simulink model "MHILSimHWImpl"  (R2024a)
settings: Solver=FixedStepDiscrete  StartTime=0.0  StopTime=2e-4  FixedStep=4e-9  RelTol=1e-3
values from neighbouring files (symbols this model uses):
  cfg = tddbl_model    [HILSimModel.m]
undefined symbols (not defined in the file or in its folder): AXI4, dt, hw, ip, Lite, xc7z020clg400
libraries: hdlBasic x1497, hdlUtilities x3, vmcUtilities x1
(part 1 of 11)
settings Model: Creator=berndorfer
settings DebuggingCC: UnconnectedInputMsg=warning  UnconnectedOutputMsg=warning  UnconnectedLineMsg=warning
settings ModelReferenceCC: EnableRefExpFcnMdlSchedulingChecks=on
settings RTWCC: GPUComputeCapability=3.5  DLArmComputeVersion=19.05

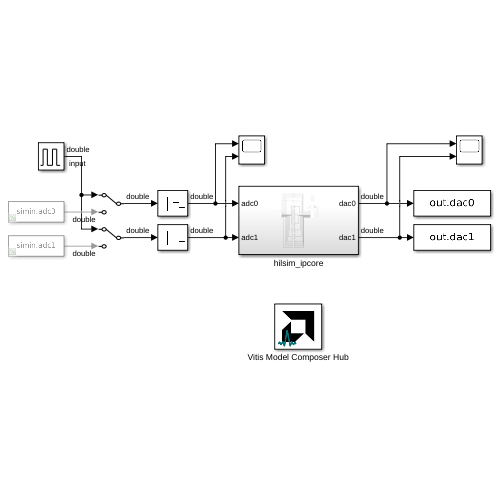
[thumbnail: Simulink's stored preview of the top-level diagram]
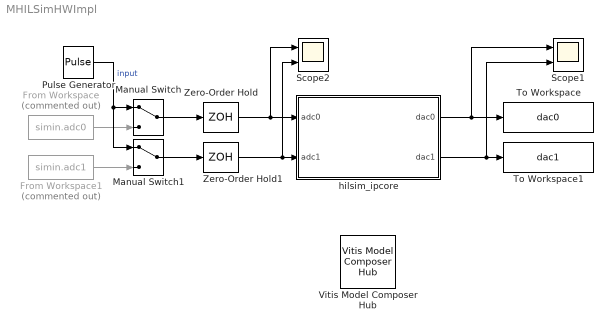
== system MHILSimHWImpl ==
  From Workspace : FromWorkspace  Commented=on  VariableName=simin.adc0
  From Workspace1 : FromWorkspace  Commented=on  VariableName=simin.adc1
  Manual Switch : ManualSwitch
  Manual Switch1 : ManualSwitch
  Pulse Generator : DiscretePulseGenerator  PulseType=Time based  Amplitude=-1  Period=2e-3  PulseWidth=4  PhaseDelay=0.05e-3
  Scope1 : Scope  NumInputPorts=2
  Scope2 : Scope  NumInputPorts=2
  To Workspace : ToWorkspace  VariableName=dac0  SaveFormat=Timeseries  SampleTime=-1
  To Workspace1 : ToWorkspace  VariableName=dac1  SaveFormat=Timeseries  SampleTime=-1
  Vitis Model Composer Hub : vmcUtilities/Vitis Model Composer Hub  Tag=genX  CodeGeneration=off  SubsystemName=hilsim_ipcore  CompilationType=HDLCompilation  SubsystemType=HDLNode  ExportTypeV2=IP Catalog  StartColumn=1  NumberOfColumns=1  TargetDirectory=./code  exportDesign=on  analyzeDesign=off  validateDesignOnHw=off  ExportType=HDL  IpVendor=xilinx.com  IpLibrary=hls  IpVersion=1.0  IpHWLanguage=Verilog  AieCompilerOptions={}  AieSimulatorOptions={}  CreateTestbench=off  TestbenchStackSize=10  RunRtlSim=off  RunCSim=off  RunAieSim=off  AieSimTimeout=50000  RunAieSimProfiling=off  LaunchVitisAnalyzer=off  PlotOutput=off  RunX86Sim=off  X86SimTimeout=10  GenHwImage=off  GenLibadfXo=on  GenHwValidationCode=off  PlatformType=Not Specified  HwSystemType=Baremetal  HwValidationTarget=hw  ProjDevice=xc7z020clg400-1  ProjDevicePart=xc7z020clg400-1  AIEType=None  SamplePeriod=-1  ClockFrequency=200  DataPathParallelism=1  xilinxfamily=zynq  part=xc7z020  speed=-1  package=clg400  directory=./code/ip/hilsim_ipcore/src  testbench=off  incr_netlist=off  synthesis_tool=Vivado  clock_wrapper=Clock Enables  dbl_ovrd=According to Block Masks  dcm_input_clock_period=10  sysclk_period=hw.t_axi_ns  simulink_period=hw.t_axi  eval_field=0  IPInfoJsonString="{\"DUTSubsystemName\":\"hilsim_ipcore\",\"HDLSubsystem\":{\"SubsystemName\":\"hilsim_ipcore\",\"IPName\":\"hilsim_ipcore\",\"IPLibrary\":\"VMC\",\"IPVendor\":\"User Company\",\"IPVersion\":\"1.0\",\"TargetDirectory\":\"./code\",\"SubsystemDir\":\"./code/ip/hilsim_ipcore\",\"FreqHz\":\"125000000\"},\"SubsystemTag\":\"HDLNode\"}"  LogFileName=/home/user/host_home/work/acin/redpitaya-hil-simulator/matlab/hilsim_lib/code/model_composer.log  NThreads=4  IPConfigFile=/tmp/vmctmp-user/10/ipconfig.json
  Zero-Order Hold : ZeroOrderHold  SampleTime=hw.t_s
  Zero-Order Hold1 : ZeroOrderHold  SampleTime=hw.t_s
  hilsim_ipcore : Subsystem
  wires:
  Zero-Order Hold1/1 -> Scope2/2, hilsim_ipcore/2(adc1)
  Zero-Order Hold/1 -> Scope2/1, hilsim_ipcore/1(adc0)
  hilsim_ipcore/1(dac0) -> To Workspace/1, Scope1/1
  hilsim_ipcore/2(dac1) -> To Workspace1/1, Scope1/2
  From Workspace/1 -> Manual Switch/2
  From Workspace1/1 -> Manual Switch1/2
  Manual Switch/1 -> Zero-Order Hold/1
  Manual Switch1/1 -> Zero-Order Hold1/1
  Pulse Generator/1 -> Manual Switch1/1, Manual Switch/1  "input"

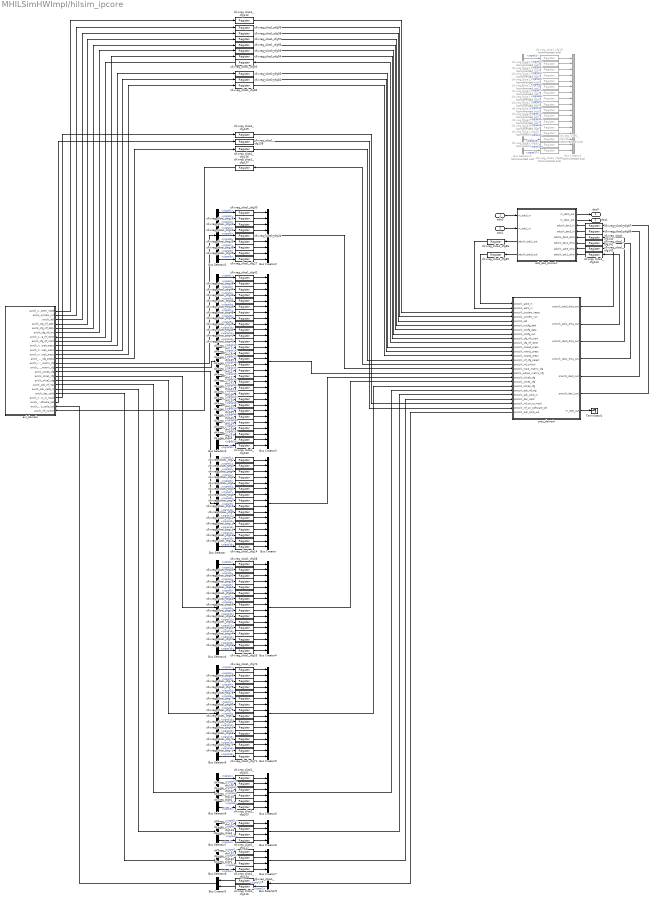
== system MHILSimHWImpl/hilsim_ipcore ==
  adc0 : Inport
  adc1 : Inport  Port=2
  Bus Creator : BusCreator  Inputs=16
  Bus Creator1 : BusCreator  Commented=on  Inputs=17
  Bus Creator2 : BusCreator  Inputs=9
  Bus Creator3 : BusCreator  Inputs=30
  Bus Creator4 : BusCreator  Inputs=16
  Bus Creator5 : BusCreator  Inputs=16
  Bus Creator6 : BusCreator  Inputs=6
  Bus Creator7 : BusCreator  Inputs=4
  Bus Creator8 : BusCreator  Inputs=4
  Bus Creator9 : BusCreator  Inputs=2
  Bus Selector : BusSelector  OutputSignals=signal1,signal2,signal3,signal4,signal5,signal6,signal7,signal8,signal9,signal10,signal11,signal12,signal13,signal14,signal15,signal16
  Bus Selector1 : BusSelector  Commented=on  OutputSignals=signal1,signal2,signal3,signal4,signal5,signal6,signal7,signal8,signal9,signal10,signal11,signal12,signal13,signal14,signal15,signal16,signal17
  Bus Selector2 : BusSelector  OutputSignals=signal1,signal2,signal3,signal4,signal5,signal6,signal7,signal8,signal9
  Bus Selector3 : BusSelector  OutputSignals=signal1,signal2,signal3,signal4,signal5,signal6,signal7,signal8,signal9,signal10,signal11,signal12,signal13,signal14,signal15,signal16,signal17,signal18,signal19,signal20,signal21,signal22,signal23,signal24,signal25,signal26,signal27,signal28,signal29,signal30
  Bus Selector4 : BusSelector  OutputSignals=signal1,signal2,signal3,signal4,signal5,signal6,signal7,signal8,signal9,signal10,signal11,signal12,signal13,signal14,signal15,signal16
  Bus Selector5 : BusSelector  OutputSignals=signal1,signal2,signal3,signal4,signal5,signal6,signal7,signal8,signal9,signal10,signal11,signal12,signal13,signal14,signal15,signal16
  Bus Selector6 : BusSelector  OutputSignals=signal1,signal2,signal3,signal4,signal5,signal6
  Bus Selector7 : BusSelector  OutputSignals=signal1,signal2,signal3,signal4
  Bus Selector8 : BusSelector  OutputSignals=signal1,signal2,signal3,signal4
  Bus Selector9 : BusSelector  OutputSignals=signal1,signal2
  Terminator2 : Terminator
  adc_dac_domain : Subsystem
      settings: PortSchema="{\"entries\":[{\"content\":{\"sides\":[{\"content\":{\"connectorIds\":[\"In1\",\"In2\",\"Out3\",\"Out4\"]},\"type\":\"ConnectorPlacement.EquallySpacedRectSide\",\"uuid\":\"3b4b5965-55e8-468b-ba12-10c3668eb49b\"},{\"content\":{\"connectorIds\":[\"Out1\",\"Out2\",\"In3\",\"In4\",\"In5\",\"In6\",\"In7\",\"In8\"],\"side\":\"RIGHT\"},\"type\":\"ConnectorPlacement.EquallySpacedRectSide\",\"uuid\":\"8bb04938-2ca8-45f3-b211-bd7f875fa19c\"},{\"content\":{\"connectorIds\":[],\"side\":\"TOP\"},\"type\":\"ConnectorPlacement.EquallySpacedRectSide\",\"uuid\":\"4c0cee75-ec1a-4ac7-a2fb-85dd83502d34\"}]},\"type\":\"ConnectorPlacement.EquallySpacedConnector\",\"uuid\":\"be0807c7-02a6-41b2-91cb-ef8260a22db3\"}],\"packageUris\":[\"http://schema.mathworks.com/mf0/Connector/R2020b\"],\"version\":\"1.0\"}"
  axi_domain : Subsystem
      settings: PortSchema="{\"entries\":[{\"content\":{\"sides\":[{\"content\":{\"connectorIds\":[]},\"type\":\"ConnectorPlacement.EquallySpacedRectSide\",\"uuid\":\"0fb9306b-ba57-4fb3-868e-1f06c1028522\"},{\"content\":{\"connectorIds\":[\"Out1\",\"Out2\",\"Out3\",\"Out4\",\"Out5\",\"Out6\",\"In1\",\"Out7\",\"Out8\",\"Out9\",\"Out10\",\"Out11\",\"Out12\",\"Out13\",\"Out14\",\"Out15\",\"Out16\",\"Out17\",\"Out18\",\"Out19\",\"Out20\",\"Out21\",\"In2\",\"In3\"],\"side\":\"RIGHT\"},\"type\":\"ConnectorPlacement.EquallySpacedRectSide\",\"uuid\":\"1b75b5fd-5ede-4f54-9992-e4e539862811\"},{\"content\":{\"connectorIds\":[],\"side\":\"TOP\"},\"type\":\"ConnectorPlacement.EquallySpacedRectSide\",\"uuid\":\"ac286cc4-83c8-4f55-8751-7af47dfb78c6\"}]},\"type\":\"ConnectorPlacement.EquallySpacedConnector\",\"uuid\":\"da69c287-1bf7-4631-a655-46508c0d45d8\"}],\"packageUris\":[\"http://schema.mathworks.com/mf0/Connector/R2020b\"],\"version\":\"1.0\"}"
  clkxreg_slice1_cfg{1..16,26..27,30..36,38..88,93..105,107..143} (126 alike) : hdlBasic/Register  init=0  rst=off  en=off  XmcBlockStatus=1  maskContainerNames=tabcontainer1  block_type=register  block_config=sysgen:Register_config
  clkxreg_slice1_cfg{17..25,28..29,37,89..92,106} (17 alike) : hdlBasic/Register  Commented=on  init=0  rst=off  en=off  XmcBlockStatus=1  maskContainerNames=tabcontainer1  block_type=register  block_config=sysgen:Register_config
  proc_domain : Subsystem
      settings: PortSchema="{\"entries\":[{\"content\":{\"sides\":[{\"content\":{\"connectorIds\":[\"In1\",\"In2\",\"In3\",\"In4\",\"In5\",\"In6\",\"In7\",\"In8\",\"In9\",\"Out8\",\"In10\",\"In11\",\"In12\",\"In13\",\"Out9\",\"In14\",\"In15\",\"In16\",\"In17\",\"In18\",\"In19\",\"In20\",\"In21\",\"In22\",\"In23\",\"Out10\"]},\"type\":\"ConnectorPlacement.EquallySpacedRectSide\",\"uuid\":\"af930565-91a0-4cb4-a54b-8373ea9a49fd\"},{\"content\":{\"connectorIds\":[\"Out1\",\"Out2\",\"Out3\",\"Out4\",\"Out5\",\"Out6\",\"Out7\"],\"side\":\"RIGHT\"},\"type\":\"ConnectorPlacement.EquallySpacedRectSide\",\"uuid\":\"8097428f-809f-46d5-8a51-08f52f31a143\"},{\"content\":{\"connectorIds\":[],\"side\":\"TOP\"},\"type\":\"ConnectorPlacement.EquallySpacedRectSide\",\"uuid\":\"c5f0461f-3302-4a3b-bb57-3345477276da\"}]},\"type\":\"ConnectorPlacement.EquallySpacedConnector\",\"uuid\":\"996f20d4-7f94-4838-9ea9-306f24b66b35\"}],\"packageUris\":[\"http://schema.mathworks.com/mf0/Connector/R2020b\"],\"version\":\"1.0\"}"
  dac0 : Outport
  dac1 : Outport  Port=2
  wires:
  axi_domain/3(axiclk_led) -> clkxreg_slice1_cfg98/1
  clkxreg_slice1_cfg98/1 -> proc_domain/5(procclk_led)
  proc_domain/7(m_leds_out) -> Terminator2/1
  axi_domain/4(axiclk_cfg_nlf_addr) -> clkxreg_slice1_cfg97/1
  axi_domain/5(axiclk_cfg_nlf_data) -> clkxreg_slice1_cfg96/1
  axi_domain/6(axiclk_cfg_nlf_we) -> clkxreg_slice1_cfg95/1
  axi_domain/7(axiclk_cfg_nlf_start) -> clkxreg_slice1_cfg94/1
  clkxreg_slice1_cfg93/1 -> axi_domain/1(axiclk_cfg_nlf_done)
  clkxreg_slice1_cfg97/1 -> proc_domain/6(procclk_lutcfg_addr)
  clkxreg_slice1_cfg96/1 -> proc_domain/7(procclk_lutcfg_data)
  clkxreg_slice1_cfg95/1 -> proc_domain/8(procclk_lutcfg_we)
  clkxreg_slice1_cfg94/1 -> proc_domain/9(procclk_cfg_nlf_start)
  proc_domain/8(procclk_cfg_nlf_done) -> clkxreg_slice1_cfg93/1
  clkxreg_slice1_cfg11/1 -> Bus Creator/12
  clkxreg_slice1_cfg12/1 -> Bus Creator/11
  clkxreg_slice1_cfg9/1 -> Bus Creator/10
  clkxreg_slice1_cfg10/1 -> Bus Creator/9
  clkxreg_slice1_cfg7/1 -> Bus Creator/8
  clkxreg_slice1_cfg8/1 -> Bus Creator/7
  clkxreg_slice1_cfg5/1 -> Bus Creator/6
  clkxreg_slice1_cfg6/1 -> Bus Creator/5
  clkxreg_slice1_cfg3/1 -> Bus Creator/4
  clkxreg_slice1_cfg4/1 -> Bus Creator/3
  clkxreg_slice1_cfg1/1 -> Bus Creator/2
  clkxreg_slice1_cfg2/1 -> Bus Creator/1
  Bus Selector/1 -> clkxreg_slice1_cfg2/1  "<signal1>"
  Bus Selector/2 -> clkxreg_slice1_cfg1/1  "<signal2>"
  Bus Selector/3 -> clkxreg_slice1_cfg4/1  "<signal3>"
  Bus Selector/4 -> clkxreg_slice1_cfg3/1  "<signal4>"
  Bus Selector/5 -> clkxreg_slice1_cfg6/1  "<signal5>"
  Bus Selector/6 -> clkxreg_slice1_cfg5/1  "<signal6>"
  Bus Selector/7 -> clkxreg_slice1_cfg8/1  "<signal7>"
  Bus Selector/8 -> clkxreg_slice1_cfg7/1  "<signal8>"
  Bus Selector/9 -> clkxreg_slice1_cfg10/1  "<signal9>"
  Bus Selector/10 -> clkxreg_slice1_cfg9/1  "<signal10>"
  Bus Selector/11 -> clkxreg_slice1_cfg12/1  "<signal11>"
  Bus Selector/12 -> clkxreg_slice1_cfg11/1  "<signal12>"
  Bus Creator/1 -> proc_domain/16(procclk_slice0_cfg)
  axi_domain/15(axiclk_slice1_cfg) -> Bus Selector4/1
  axi_domain/2(axiclk_system_run) -> clkxreg_slice1_cfg99/1
  clkxreg_slice1_cfg99/1 -> proc_domain/4(procclk_system_run)
  clkxreg_slice1_cfg13/1 -> Bus Creator/13
  clkxreg_slice1_cfg16/1 -> Bus Creator/14
  clkxreg_slice1_cfg15/1 -> Bus Creator/15
  clkxreg_slice1_cfg14/1 -> Bus Creator/16
  Bus Selector/13 -> clkxreg_slice1_cfg13/1  "<signal13>"
  Bus Selector/14 -> clkxreg_slice1_cfg16/1  "<signal14>"
  Bus Selector/15 -> clkxreg_slice1_cfg15/1  "<signal15>"
  Bus Selector/16 -> clkxreg_slice1_cfg14/1  "<signal16>"
  clkxreg_slice1_cfg18/1 -> Bus Creator1/9
  clkxreg_slice1_cfg24/1 -> Bus Creator1/8
  clkxreg_slice1_cfg25/1 -> Bus Creator1/7
  clkxreg_slice1_cfg22/1 -> Bus Creator1/6
  clkxreg_slice1_cfg23/1 -> Bus Creator1/5
  clkxreg_slice1_cfg20/1 -> Bus Creator1/4
  clkxreg_slice1_cfg21/1 -> Bus Creator1/3
  clkxreg_slice1_cfg17/1 -> Bus Creator1/2
  clkxreg_slice1_cfg19/1 -> Bus Creator1/1
  Bus Selector1/9 -> clkxreg_slice1_cfg18/1  "<signal9>"
  Bus Selector1/8 -> clkxreg_slice1_cfg24/1  "<signal8>"
  Bus Selector1/7 -> clkxreg_slice1_cfg25/1  "<signal7>"
  Bus Selector1/6 -> clkxreg_slice1_cfg22/1  "<signal6>"
  Bus Selector1/5 -> clkxreg_slice1_cfg23/1  "<signal5>"
  Bus Selector1/4 -> clkxreg_slice1_cfg20/1  "<signal4>"
  Bus Selector1/3 -> clkxreg_slice1_cfg21/1  "<signal3>"
  Bus Selector1/2 -> clkxreg_slice1_cfg17/1  "<signal2>"
  Bus Selector1/1 -> clkxreg_slice1_cfg19/1  "<signal1>"
  clkxreg_slice1_cfg136/1 -> proc_domain/13(procclk_nlf_cfg_select)
  Bus Selector2/1 -> clkxreg_slice1_cfg30/1  "<signal1>"
  Bus Selector2/2 -> clkxreg_slice1_cfg26/1  "<signal2>"
  Bus Selector2/3 -> clkxreg_slice1_cfg32/1  "<signal3>"
  Bus Selector2/4 -> clkxreg_slice1_cfg31/1  "<signal4>"
  Bus Selector2/5 -> clkxreg_slice1_cfg34/1  "<signal5>"
  Bus Selector2/6 -> clkxreg_slice1_cfg33/1  "<signal6>"
  Bus Selector2/7 -> clkxreg_slice1_cfg36/1  "<signal7>"
  Bus Selector2/8 -> clkxreg_slice1_cfg35/1  "<signal8>"
  Bus Selector2/9 -> clkxreg_slice1_cfg27/1  "<signal9>"
  clkxreg_slice1_cfg30/1 -> Bus Creator2/1
  clkxreg_slice1_cfg26/1 -> Bus Creator2/2
  clkxreg_slice1_cfg32/1 -> Bus Creator2/3
  clkxreg_slice1_cfg31/1 -> Bus Creator2/4
  clkxreg_slice1_cfg34/1 -> Bus Creator2/5
  clkxreg_slice1_cfg33/1 -> Bus Creator2/6
  clkxreg_slice1_cfg36/1 -> Bus Creator2/7
  clkxreg_slice1_cfg35/1 -> Bus Creator2/8
  clkxreg_slice1_cfg27/1 -> Bus Creator2/9
  Bus Creator2/1 -> proc_domain/14(procclk_input_matrix_cfg)
  Bus Selector3/8 -> clkxreg_slice1_cfg47/1  "<signal8>"
  Bus Selector3/10 -> clkxreg_slice1_cfg49/1  "<signal10>"
  Bus Selector3/12 -> clkxreg_slice1_cfg40/1  "<signal12>"
  clkxreg_slice1_cfg41/1 -> Bus Creator3/11
  Bus Selector3/4 -> clkxreg_slice1_cfg43/1  "<signal4>"
  Bus Selector3/7 -> clkxreg_slice1_cfg48/1  "<signal7>"
  Bus Selector3/9 -> clkxreg_slice1_cfg39/1  "<signal9>"
  clkxreg_slice1_cfg42/1 -> Bus Creator3/1
  clkxreg_slice1_cfg45/1 -> Bus Creator3/6
  clkxreg_slice1_cfg44/1 -> Bus Creator3/3
  clkxreg_slice1_cfg48/1 -> Bus Creator3/7
  clkxreg_slice1_cfg43/1 -> Bus Creator3/4
  clkxreg_slice1_cfg40/1 -> Bus Creator3/12
  clkxreg_slice1_cfg46/1 -> Bus Creator3/5
  Bus Selector3/2 -> clkxreg_slice1_cfg38/1  "<signal2>"
  clkxreg_slice1_cfg38/1 -> Bus Creator3/2
  clkxreg_slice1_cfg39/1 -> Bus Creator3/9
  Bus Selector3/3 -> clkxreg_slice1_cfg44/1  "<signal3>"
  Bus Selector3/5 -> clkxreg_slice1_cfg46/1  "<signal5>"
  Bus Selector3/11 -> clkxreg_slice1_cfg41/1  "<signal11>"
  clkxreg_slice1_cfg47/1 -> Bus Creator3/8
  clkxreg_slice1_cfg49/1 -> Bus Creator3/10
  Bus Selector3/6 -> clkxreg_slice1_cfg45/1  "<signal6>"
  Bus Selector3/1 -> clkxreg_slice1_cfg42/1  "<signal1>"
  Bus Creator3/1 -> proc_domain/15(adcclk_output_matrix_cfg)
  Bus Selector4/14 -> clkxreg_slice1_cfg57/1  "<signal14>"
  Bus Selector4/5 -> clkxreg_slice1_cfg62/1  "<signal5>"
  clkxreg_slice1_cfg65/1 -> Bus Creator4/10
  clkxreg_slice1_cfg52/1 -> Bus Creator4/12
  clkxreg_slice1_cfg62/1 -> Bus Creator4/5
  Bus Selector4/16 -> clkxreg_slice1_cfg55/1  "<signal16>"
  Bus Selector4/3 -> clkxreg_slice1_cfg60/1  "<signal3>"
  clkxreg_slice1_cfg61/1 -> Bus Creator4/6
  Bus Selector4/4 -> clkxreg_slice1_cfg59/1  "<signal4>"
  clkxreg_slice1_cfg58/1 -> Bus Creator4/1
  Bus Selector4/10 -> clkxreg_slice1_cfg65/1  "<signal10>"
  Bus Selector4/7 -> clkxreg_slice1_cfg64/1  "<signal7>"
  clkxreg_slice1_cfg51/1 -> Bus Creator4/9
  clkxreg_slice1_cfg57/1 -> Bus Creator4/14
  Bus Selector4/8 -> clkxreg_slice1_cfg63/1  "<signal8>"
  Bus Selector4/13 -> clkxreg_slice1_cfg54/1  "<signal13>"
  Bus Selector4/9 -> clkxreg_slice1_cfg51/1  "<signal9>"
  clkxreg_slice1_cfg50/1 -> Bus Creator4/2
  clkxreg_slice1_cfg64/1 -> Bus Creator4/7
  Bus Selector4/11 -> clkxreg_slice1_cfg53/1  "<signal11>"
  Bus Selector4/15 -> clkxreg_slice1_cfg56/1  "<signal15>"
  Bus Selector4/12 -> clkxreg_slice1_cfg52/1  "<signal12>"
  clkxreg_slice1_cfg56/1 -> Bus Creator4/15
  clkxreg_slice1_cfg59/1 -> Bus Creator4/4
  clkxreg_slice1_cfg54/1 -> Bus Creator4/13
  clkxreg_slice1_cfg60/1 -> Bus Creator4/3
  clkxreg_slice1_cfg53/1 -> Bus Creator4/11
  clkxreg_slice1_cfg55/1 -> Bus Creator4/16
  Bus Selector4/2 -> clkxreg_slice1_cfg50/1  "<signal2>"
  Bus Selector4/1 -> clkxreg_slice1_cfg58/1  "<signal1>"
  clkxreg_slice1_cfg63/1 -> Bus Creator4/8
  Bus Selector4/6 -> clkxreg_slice1_cfg61/1  "<signal6>"
  Bus Selector5/14 -> clkxreg_slice1_cfg73/1  "<signal14>"
  Bus Selector5/5 -> clkxreg_slice1_cfg78/1  "<signal5>"
  clkxreg_slice1_cfg81/1 -> Bus Creator5/10
  clkxreg_slice1_cfg68/1 -> Bus Creator5/12
  clkxreg_slice1_cfg78/1 -> Bus Creator5/5
  Bus Selector5/16 -> clkxreg_slice1_cfg71/1  "<signal16>"
  Bus Selector5/3 -> clkxreg_slice1_cfg76/1  "<signal3>"
  clkxreg_slice1_cfg77/1 -> Bus Creator5/6
  Bus Selector5/4 -> clkxreg_slice1_cfg75/1  "<signal4>"
  clkxreg_slice1_cfg74/1 -> Bus Creator5/1
  Bus Selector5/10 -> clkxreg_slice1_cfg81/1  "<signal10>"
  Bus Selector5/7 -> clkxreg_slice1_cfg80/1  "<signal7>"
  clkxreg_slice1_cfg67/1 -> Bus Creator5/9
  clkxreg_slice1_cfg73/1 -> Bus Creator5/14
  Bus Selector5/8 -> clkxreg_slice1_cfg79/1  "<signal8>"
  Bus Selector5/13 -> clkxreg_slice1_cfg70/1  "<signal13>"
  Bus Selector5/9 -> clkxreg_slice1_cfg67/1  "<signal9>"
  clkxreg_slice1_cfg66/1 -> Bus Creator5/2
  clkxreg_slice1_cfg80/1 -> Bus Creator5/7
  Bus Selector5/11 -> clkxreg_slice1_cfg69/1  "<signal11>"
  Bus Selector5/15 -> clkxreg_slice1_cfg72/1  "<signal15>"
  Bus Selector5/12 -> clkxreg_slice1_cfg68/1  "<signal12>"
  clkxreg_slice1_cfg72/1 -> Bus Creator5/15
  clkxreg_slice1_cfg75/1 -> Bus Creator5/4
  clkxreg_slice1_cfg70/1 -> Bus Creator5/13
  clkxreg_slice1_cfg76/1 -> Bus Creator5/3
  clkxreg_slice1_cfg69/1 -> Bus Creator5/11
  clkxreg_slice1_cfg71/1 -> Bus Creator5/16
  Bus Selector5/2 -> clkxreg_slice1_cfg66/1  "<signal2>"
  Bus Selector5/1 -> clkxreg_slice1_cfg74/1  "<signal1>"
  clkxreg_slice1_cfg79/1 -> Bus Creator5/8
  Bus Selector5/6 -> clkxreg_slice1_cfg77/1  "<signal6>"
  Bus Creator5/1 -> proc_domain/18(procclk_slice2_cfg)
  clkxreg_slice1_cfg83/1 -> proc_domain/10(procclk_noise0_presc)
  clkxreg_slice1_cfg82/1 -> proc_domain/11(procclk_noise1_presc)
  clkxreg_slice1_cfg84/1 -> proc_domain/12(procclk_noise2_presc)
  axi_domain/11(axiclk_nlf_cfg_select) -> clkxreg_slice1_cfg136/1
  axi_domain/12(axiclk_input_matrix_cfg) -> Bus Selector2/1
  axi_domain/13(axiclk_output_matrix_cfg) -> Bus Selector3/1
  axi_domain/14(axiclk_slice0_cfg) -> Bus Selector/1
  axi_domain/16(axiclk_slice2_cfg) -> Bus Selector5/1
  axi_domain/8(axiclk_noise0_presc) -> clkxreg_slice1_cfg83/1
  axi_domain/9(axiclk_noise1_presc) -> clkxreg_slice1_cfg82/1
  axi_domain/10(axiclk_noise2_presc) -> clkxreg_slice1_cfg84/1
  adc0/1 -> adc_dac_domain/1(m_adc0_in)
  adc1/1 -> adc_dac_domain/2(m_adc1_in)
  adc_dac_domain/3(adcclk_adc1_out) -> clkxreg_slice1_cfg86/1
  adc_dac_domain/4(adcclk_adc0_out) -> clkxreg_slice1_cfg85/1
  clkxreg_slice1_cfg85/1 -> proc_domain/1(procclk_adc0_in)
  clkxreg_slice1_cfg86/1 -> proc_domain/2(procclk_adc1_in)
  clkxreg_slice1_cfg88/1 -> adc_dac_domain/4(adcclk_dac0_in)
  clkxreg_slice1_cfg87/1 -> adc_dac_domain/3(adcclk_dac1_in)
  adc_dac_domain/1(m_dac0_out) -> dac0/1
  adc_dac_domain/2(m_dac1_out) -> dac1/1
  proc_domain/5(procclk_dac0_out) -> clkxreg_slice1_cfg88/1
  proc_domain/6(procclk_dac1_out) -> clkxreg_slice1_cfg87/1
  Bus Creator4/1 -> proc_domain/17(procclk_slice1_cfg)
  clkxreg_slice1_cfg90/1 -> Bus Creator1/10
  clkxreg_slice1_cfg92/1 -> Bus Creator1/11
  clkxreg_slice1_cfg91/1 -> Bus Creator1/12
  clkxreg_slice1_cfg89/1 -> Bus Creator1/13
  Bus Selector1/10 -> clkxreg_slice1_cfg90/1  "<signal10>"
  Bus Selector1/11 -> clkxreg_slice1_cfg92/1  "<signal11>"
  Bus Selector1/12 -> clkxreg_slice1_cfg91/1  "<signal12>"
  Bus Selector1/13 -> clkxreg_slice1_cfg89/1  "<signal13>"
  Bus Selector6/6 -> clkxreg_slice1_cfg103/1  "<signal6>"
  Bus Selector6/5 -> clkxreg_slice1_cfg104/1  "<signal5>"
  Bus Selector6/4 -> clkxreg_slice1_cfg105/1  "<signal4>"
  Bus Selector6/3 -> clkxreg_slice1_cfg102/1  "<signal3>"
  Bus Selector6/2 -> clkxreg_slice1_cfg100/1  "<signal2>"
  Bus Selector6/1 -> clkxreg_slice1_cfg101/1  "<signal1>"
  clkxreg_slice1_cfg101/1 -> Bus Creator6/1
  clkxreg_slice1_cfg100/1 -> Bus Creator6/2
  clkxreg_slice1_cfg102/1 -> Bus Creator6/3
  clkxreg_slice1_cfg105/1 -> Bus Creator6/4
  clkxreg_slice1_cfg104/1 -> Bus Creator6/5
  clkxreg_slice1_cfg103/1 -> Bus Creator6/6
  Bus Creator6/1 -> proc_domain/19(procclk_adc_nlf_cfg)
  axi_domain/17(axiclk_adc_nlf_cfg) -> Bus Selector6/1
  clkxreg_slice1_cfg112/1 -> proc_domain/3(procclk_system_reset)
  axi_domain/1(axiclk_system_reset) -> clkxreg_slice1_cfg112/1
  clkxreg_slice1_cfg114/1 -> Bus Creator8/1
  clkxreg_slice1_cfg113/1 -> Bus Creator8/2
  Bus Selector7/1 -> clkxreg_slice1_cfg114/1  "<signal1>"
  Bus Selector7/2 -> clkxreg_slice1_cfg113/1  "<signal2>"
  axi_domain/18(axiclk_adc_calib_in) -> Bus Selector7/1
  clkxreg_slice1_cfg115/1 -> Bus Creator9/1
  clkxreg_slice1_cfg116/1 -> Bus Creator9/2
  Bus Selector9/1 -> clkxreg_slice1_cfg115/1  "<signal1>"
  Bus Selector9/2 -> clkxreg_slice1_cfg116/1  "<signal2>"
  Bus Creator9/1 -> axi_domain/2(axiclk_adc_calib_out)
  Bus Creator8/1 -> proc_domain/20(procclk_adc_calib_in)
  proc_domain/10(procclk_adc_calib_out) -> Bus Selector9/1
  Bus Selector7/3 -> clkxreg_slice1_cfg118/1  "<signal3>"
  Bus Selector7/4 -> clkxreg_slice1_cfg117/1  "<signal4>"
  clkxreg_slice1_cfg118/1 -> Bus Creator8/3
  clkxreg_slice1_cfg117/1 -> Bus Creator8/4
  Bus Selector1/14 -> clkxreg_slice1_cfg29/1  "<signal14>"
  Bus Selector1/15 -> clkxreg_slice1_cfg106/1  "<signal15>"
  Bus Selector1/16 -> clkxreg_slice1_cfg37/1  "<signal16>"
  Bus Selector1/17 -> clkxreg_slice1_cfg28/1  "<signal17>"
  clkxreg_slice1_cfg28/1 -> Bus Creator1/17
  clkxreg_slice1_cfg37/1 -> Bus Creator1/16
  clkxreg_slice1_cfg106/1 -> Bus Creator1/15
  clkxreg_slice1_cfg29/1 -> Bus Creator1/14
  Bus Selector3/13 -> clkxreg_slice1_cfg111/1  "<signal13>"
  Bus Selector3/14 -> clkxreg_slice1_cfg107/1  "<signal14>"
  Bus Selector3/15 -> clkxreg_slice1_cfg120/1  "<signal15>"
  Bus Selector3/16 -> clkxreg_slice1_cfg119/1  "<signal16>"
  Bus Selector3/17 -> clkxreg_slice1_cfg122/1  "<signal17>"
  Bus Selector3/18 -> clkxreg_slice1_cfg121/1  "<signal18>"
  Bus Selector3/19 -> clkxreg_slice1_cfg124/1  "<signal19>"
  Bus Selector3/20 -> clkxreg_slice1_cfg123/1  "<signal20>"
  Bus Selector3/21 -> clkxreg_slice1_cfg108/1  "<signal21>"
  Bus Selector3/22 -> clkxreg_slice1_cfg125/1  "<signal22>"
  Bus Selector3/23 -> clkxreg_slice1_cfg110/1  "<signal23>"
  Bus Selector3/24 -> clkxreg_slice1_cfg109/1  "<signal24>"
  Bus Selector3/25 -> clkxreg_slice1_cfg126/1  "<signal25>"
  Bus Selector3/26 -> clkxreg_slice1_cfg129/1  "<signal26>"
  Bus Selector3/27 -> clkxreg_slice1_cfg128/1  "<signal27>"
  Bus Selector3/28 -> clkxreg_slice1_cfg127/1  "<signal28>"
  Bus Selector3/29 -> clkxreg_slice1_cfg131/1  "<signal29>"
  Bus Selector3/30 -> clkxreg_slice1_cfg130/1  "<signal30>"
  clkxreg_slice1_cfg111/1 -> Bus Creator3/13
  clkxreg_slice1_cfg107/1 -> Bus Creator3/14
  clkxreg_slice1_cfg120/1 -> Bus Creator3/15
  clkxreg_slice1_cfg119/1 -> Bus Creator3/16
  clkxreg_slice1_cfg122/1 -> Bus Creator3/17
  clkxreg_slice1_cfg121/1 -> Bus Creator3/18
  clkxreg_slice1_cfg124/1 -> Bus Creator3/19
  clkxreg_slice1_cfg123/1 -> Bus Creator3/20
  clkxreg_slice1_cfg108/1 -> Bus Creator3/21
  clkxreg_slice1_cfg125/1 -> Bus Creator3/22
  clkxreg_slice1_cfg110/1 -> Bus Creator3/23
  clkxreg_slice1_cfg109/1 -> Bus Creator3/24
  clkxreg_slice1_cfg126/1 -> Bus Creator3/25
  clkxreg_slice1_cfg129/1 -> Bus Creator3/26
  clkxreg_slice1_cfg128/1 -> Bus Creator3/27
  clkxreg_slice1_cfg127/1 -> Bus Creator3/28
  clkxreg_slice1_cfg131/1 -> Bus Creator3/29
  clkxreg_slice1_cfg130/1 -> Bus Creator3/30
  clkxreg_slice1_cfg135/1 -> Bus Creator7/3
  clkxreg_slice1_cfg133/1 -> Bus Creator7/1
  Bus Selector8/4 -> clkxreg_slice1_cfg134/1  "<signal4>"
  Bus Selector8/3 -> clkxreg_slice1_cfg135/1  "<signal3>"
  clkxreg_slice1_cfg132/1 -> Bus Creator7/2
  Bus Selector8/1 -> clkxreg_slice1_cfg133/1  "<signal1>"
  clkxreg_slice1_cfg134/1 -> Bus Creator7/4
  Bus Selector8/2 -> clkxreg_slice1_cfg132/1  "<signal2>"
  axi_domain/19(axiclk_dac_calib) -> Bus Selector8/1
  Bus Creator7/1 -> proc_domain/21(procclk_dac_calib)
  proc_domain/9(procclk_nlf_switch) -> clkxreg_slice1_cfg137/1
  clkxreg_slice1_cfg137/1 -> axi_domain/3(axiclk_nlf_switch)
  axi_domain/20(axiclk_nlf_sw_io_mask) -> clkxreg_slice1_cfg139/1
  axi_domain/21(axiclk_nlf_sw_software_sel) -> clkxreg_slice1_cfg138/1
  clkxreg_slice1_cfg139/1 -> proc_domain/22(procclk_nlf_sw_io_mask)
  clkxreg_slice1_cfg138/1 -> proc_domain/23(procclk_nlf_sw_software_sel)
  clkxreg_slice1_cfg140/1 -> adc_dac_domain/5(adcclk_dac0_dma)
  clkxreg_slice1_cfg141/1 -> adc_dac_domain/6(adcclk_dac1_dma)
  clkxreg_slice1_cfg142/1 -> adc_dac_domain/7(adcclk_adc0_dma)
  clkxreg_slice1_cfg143/1 -> adc_dac_domain/8(adcclk_adc1_dma)
  proc_domain/4(procclk_dac1_dma_out) -> clkxreg_slice1_cfg141/1
  proc_domain/3(procclk_dac0_dma_out) -> clkxreg_slice1_cfg140/1
  proc_domain/2(procclk_adc1_dma_out) -> clkxreg_slice1_cfg143/1
  proc_domain/1(procclk_adc0_dma_out) -> clkxreg_slice1_cfg142/1

== system MHILSimHWImpl/hilsim_ipcore/adc_dac_domain ==
  m_adc0_in : Inport
  m_adc1_in : Inport  Port=2
  adcclk_dac1_in : Inport  Port=3
  adcclk_dac0_in : Inport  Port=4
  adcclk_dac0_dma : Inport  Port=5
  adcclk_dac1_dma : Inport  Port=6
  adcclk_adc0_dma : Inport  Port=7
  adcclk_adc1_dma : Inport  Port=8
  Concat : hdlBasic/Concat  num_inputs=2  XmcBlockStatus=1  maskContainerNames=group1  block_type=concat  block_config=sysgen:Concat_config
  Constant7 : hdlBasic/Constant  const=0  gui_display_data_type=Fixed-point  arith_type=Unsigned  n_bits=1  bin_pt=0  preci_type=Single  exp_width=8  frac_width=24  explicit_period=off  period=1  XmcBlockStatus=1  maskContainerNames=tabcontainer1  block_type=constant  block_config=sysgen:Constant_config
  Terminator{3..6} (4 alike) : Terminator
  adc_ch0_in : hdlBasic/Gateway In  gui_display_data_type=Fixed-point  arith_type=Signed (2's comp)  n_bits=dt.adc.sz  bin_pt=dt.adc.bin  preci_type=Single  exp_width=8  frac_width=24  rows=1  columns=1  quantization="Round  (unbiased: +/- Inf)"  overflow=Saturate  period=hw.t_adc  UseAsADC=off  ADCChannel='1'  interface=None  automatic_assignment=on  address_offset=hex2dec('00')  intf_name=''  intf_description=''  default_value=0  timing_constraint=None  locs_specified=off  LOCs={}  io_standard={}  inherit_from_input=off  hdl_port=on  XmcBlockStatus=1  maskContainerNames=group4  block_type=gatewayin  block_config=sysgen:gateway_in_config  block_width_w=590  block_height_w=620  block_width=640  block_height=850
  adc_ch1_in : hdlBasic/Gateway In  gui_display_data_type=Fixed-point  arith_type=Signed (2's comp)  n_bits=dt.adc.sz  bin_pt=dt.adc.bin  preci_type=Single  exp_width=8  frac_width=24  rows=1  columns=1  quantization="Round  (unbiased: +/- Inf)"  overflow=Saturate  period=hw.t_adc  UseAsADC=off  ADCChannel='1'  interface=None  automatic_assignment=on  address_offset=hex2dec('00')  intf_name=''  intf_description=''  default_value=0  timing_constraint=None  locs_specified=off  LOCs={}  io_standard={}  inherit_from_input=off  hdl_port=on  XmcBlockStatus=1  maskContainerNames=group4  block_type=gatewayin  block_config=sysgen:gateway_in_config  block_width_w=590  block_height_w=620  block_width=640  block_height=850
  cast_adc0_to_slice : hdlBasic/Convert  gui_display_data_type=Fixed-point  arith_type=Signed (2's comp)  n_bits=dt.slice.sz  bin_pt=dt.slice.bin  float_type=Single  exp_bits=8  fraction_bits=24  quantization=Truncate  overflow=Wrap  en=off  latency=0  pipeline=off  XmcBlockStatus=1  maskContainerNames=group2  block_type=convert  block_config=sysgen:Convert_config  block_width=595  block_height=885
  cast_adc1_to_slice : hdlBasic/Convert  gui_display_data_type=Fixed-point  arith_type=Signed (2's comp)  n_bits=dt.slice.sz  bin_pt=dt.slice.bin  float_type=Single  exp_bits=8  fraction_bits=24  quantization=Truncate  overflow=Wrap  en=off  latency=0  pipeline=off  XmcBlockStatus=1  maskContainerNames=group2  block_type=convert  block_config=sysgen:Convert_config  block_width=595  block_height=885
  cast_dac0 : hdlBasic/Convert  gui_display_data_type=Fixed-point  arith_type=Signed (2's comp)  n_bits=dt.adc.sz  bin_pt=dt.adc.bin  float_type=Single  exp_bits=8  fraction_bits=24  quantization=Truncate  overflow=Wrap  en=off  latency=0  pipeline=off  XmcBlockStatus=1  maskContainerNames=group2  block_type=convert  block_config=sysgen:Convert_config  block_width=595  block_height=885
  cast_dac1 : hdlBasic/Convert  gui_display_data_type=Fixed-point  arith_type=Signed (2's comp)  n_bits=dt.adc.sz  bin_pt=dt.adc.bin  float_type=Single  exp_bits=8  fraction_bits=24  quantization=Truncate  overflow=Wrap  en=off  latency=0  pipeline=off  XmcBlockStatus=1  maskContainerNames=group2  block_type=convert  block_config=sysgen:Convert_config  block_width=595  block_height=885
  cast_dma{,1..3} (4 alike) : hdlBasic/Convert  gui_display_data_type=Fixed-point  arith_type=Signed (2's comp)  n_bits=dt.dma.sz  bin_pt=dt.dma.bin  float_type=Single  exp_bits=8  fraction_bits=24  quantization=Truncate  overflow=Wrap  en=off  latency=0  pipeline=off  XmcBlockStatus=1  maskContainerNames=group2  block_type=convert  block_config=sysgen:Convert_config  block_width=595  block_height=885
  dac_ch0_out : hdlBasic/Gateway Out  inherit_from_input=off  hdl_port=on  rows=1  columns=1  UseAsDAC=off  DACChannel='1'  interface=None  automatic_assignment=on  address_offset=hex2dec('00')  intf_name=''  intf_description=''  timing_constraint=None  locs_specified=off  LOCs={}  io_standard={}  XmcBlockStatus=1  maskContainerNames=group4  block_type=gatewayout  block_config=sysgen:gateway_out_config  block_width_w=590  block_height_w=620  block_width=620  block_height=750
  dac_ch1_out : hdlBasic/Gateway Out  inherit_from_input=off  hdl_port=on  rows=1  columns=1  UseAsDAC=off  DACChannel='1'  interface=None  automatic_assignment=on  address_offset=hex2dec('00')  intf_name=''  intf_description=''  timing_constraint=None  locs_specified=off  LOCs={}  io_standard={}  XmcBlockStatus=1  maskContainerNames=group4  block_type=gatewayout  block_config=sysgen:gateway_out_config  block_width_w=590  block_height_w=620  block_width=620  block_height=750
  dma_ch1_out : hdlBasic/Gateway Out  inherit_from_input=off  hdl_port=on  rows=1  columns=1  UseAsDAC=off  DACChannel='1'  interface=None  automatic_assignment=on  address_offset=hex2dec('00')  intf_name=''  intf_description=''  timing_constraint=None  locs_specified=off  LOCs={}  io_standard={}  XmcBlockStatus=1  maskContainerNames=group4  block_type=gatewayout  block_config=sysgen:gateway_out_config  block_width_w=590  block_height_w=620  block_width=620  block_height=750
  dma_ch2h_out : hdlBasic/Gateway Out  inherit_from_input=off  hdl_port=on  rows=1  columns=1  UseAsDAC=off  DACChannel='1'  interface=None  automatic_assignment=on  address_offset=hex2dec('00')  intf_name=''  intf_description=''  timing_constraint=None  locs_specified=off  LOCs={}  io_standard={}  XmcBlockStatus=1  maskContainerNames=group4  block_type=gatewayout  block_config=sysgen:gateway_out_config  block_width_w=590  block_height_w=620  block_width=620  block_height=750
  dma_ch2l_out : hdlBasic/Gateway Out  inherit_from_input=off  hdl_port=on  rows=1  columns=1  UseAsDAC=off  DACChannel='1'  interface=None  automatic_assignment=on  address_offset=hex2dec('00')  intf_name=''  intf_description=''  timing_constraint=None  locs_specified=off  LOCs={}  io_standard={}  XmcBlockStatus=1  maskContainerNames=group4  block_type=gatewayout  block_config=sysgen:gateway_out_config  block_width_w=590  block_height_w=620  block_width=620  block_height=750
  dma_trigger_out : hdlBasic/Gateway Out  inherit_from_input=off  hdl_port=on  rows=1  columns=1  UseAsDAC=off  DACChannel='1'  interface=None  automatic_assignment=on  address_offset=hex2dec('00')  intf_name=''  intf_description=''  timing_constraint=None  locs_specified=off  LOCs={}  io_standard={}  XmcBlockStatus=1  maskContainerNames=group4  block_type=gatewayout  block_config=sysgen:gateway_out_config  block_width_w=590  block_height_w=620  block_width=620  block_height=750
  reint_u{1..3,16} (4 alike) : hdlBasic/Reinterpret  force_arith_type=on  arith_type=Unsigned  force_bin_pt=on  bin_pt=0  XmcBlockStatus=1  maskContainerNames=group1  block_type=reinterpret  block_config=sysgen:Reinterpret_config
  m_dac0_out : Outport
  m_dac1_out : Outport  Port=2
  adcclk_adc1_out : Outport  Port=3
  adcclk_adc0_out : Outport  Port=4
  wires:
  adc_ch0_in/1 -> cast_adc0_to_slice/1
  adc_ch1_in/1 -> cast_adc1_to_slice/1
  m_adc0_in/1 -> adc_ch0_in/1
  m_adc1_in/1 -> adc_ch1_in/1
  cast_adc0_to_slice/1 -> adcclk_adc0_out/1
  cast_adc1_to_slice/1 -> adcclk_adc1_out/1
  cast_dac0/1 -> dac_ch0_out/1
  cast_dac1/1 -> dac_ch1_out/1
  adcclk_dac0_in/1 -> cast_dac0/1
  adcclk_dac1_in/1 -> cast_dac1/1
  dac_ch0_out/1 -> m_dac0_out/1
  dac_ch1_out/1 -> m_dac1_out/1
  dma_ch2h_out/1 -> Terminator4/1
  dma_ch1_out/1 -> Terminator3/1
  dma_ch2l_out/1 -> Terminator5/1
  dma_trigger_out/1 -> Terminator6/1
  Constant7/1 -> dma_trigger_out/1
  adcclk_dac0_dma/1 -> cast_dma1/1
  adcclk_dac1_dma/1 -> cast_dma/1
  cast_dma/1 -> reint_u16/1
  Concat/1 -> dma_ch1_out/1
  cast_dma1/1 -> reint_u1/1
  reint_u16/1 -> Concat/1
  reint_u1/1 -> Concat/2
  cast_dma3/1 -> reint_u2/1
  cast_dma2/1 -> reint_u3/1
  adcclk_adc0_dma/1 -> cast_dma2/1
  adcclk_adc1_dma/1 -> cast_dma3/1
  reint_u3/1 -> dma_ch2l_out/1
  reint_u2/1 -> dma_ch2h_out/1
